simulink model "Code_2DoF_Simulation_myori"  (R2022b)
settings: Solver=ode4  StartTime=0  StopTime=32  FixedStep=0.0025  MaxStep=0.005  MinStep=0.001  RelTol=0.5
settings Model: Creator=hp  LastModifiedBy=33093
settings SolverCC: AlgebraicLoopSolver=TrustRegion
settings DataIOCC: ExternalInput=untitled.getElement(1),[],[],[],[],[],[],[],[],[],[],[],[],[],[],[],[],[],[]  SaveFormat=Array  SignalLoggingSaveFormat=ModelDataLogs  ReturnWorkspaceOutputs=off  SignalLoggingName=sigsOut
settings OptimizationCC: DefaultParameterBehavior=Inlined  UseDivisionForNetSlopeComputation=on  UseFloatMulNetSlope=on  InlineInvariantSignals=on  PassReuseOutputArgsAs=Individual arguments  ExpressionDepthLimit=2147483647  ZeroExternalMemoryAtStartup=off  ZeroInternalMemoryAtStartup=off  NoFixptDivByZeroProtection=on  EfficientFloat2IntCast=on  LifeSpan=1  EfficientTunableParamExpr=on
settings DebuggingCC: SaveWithParameterizedLinksMsg=none  UnderspecifiedInitializationDetection=Classic  MergeDetectMultiDrivingBlocksExec=none  SignalResolutionControl=TryResolveAllWithWarning  MultiTaskDSMMsg=warning  MultiTaskCondExecSysMsg=none  MultiTaskRateTransMsg=warning  ParameterTunabilityLossMsg=error  FcnCallInpInsideContextMsg=warning  UnconnectedInputMsg=warning  UnconnectedOutputMsg=warning  UnconnectedLineMsg=warning  StateNameClashWarn=warning  SFUnexpectedBacktrackingDiag=warning  SFNoUnconditionalDefaultTransitionDiag=warning  SFExecutionAtInitializationDiag=none  SFMachineParentedDataDiag=warning  ArithmeticOperatorsInVariantConditions=warning
settings HardwareCC: TargetBitPerPointer=64  TargetBitPerSizeT=64  TargetBitPerPtrDiffT=64  TargetLongLongMode=on  TargetIntDivRoundTo=Zero  TargetEndianess=LittleEndian  TargetWordSize=64  TargetHWDeviceType=MATLAB Host  ProdEqTarget=off
settings ModelReferenceCC: EnableRefExpFcnMdlSchedulingChecks=on  PropagateSignalLabelsOutOfModel=off
settings SFSimCC: SimUseLocalCustomCode=off  MATLABDynamicMemAlloc=off  CustomCodeUndefinedFunction=UseInterfaceOnly
settings RTWCC: Description=Embedded Coder  SystemTargetFile=ert.tlc  TemplateMakefile=ert_default_tmf  GenerateReport=on  RTWUseLocalCustomCode=off  IncludeHyperlinkInReport=on  LaunchReport=on  GenerateTraceInfo=on  GenerateTraceReport=on  GenerateTraceReportSl=on  GenerateTraceReportSf=on  GenerateTraceReportEml=on  GenerateCodeMetricsReport=on
settings CodeAppCC: ForceParamTrailComments=on  IgnoreCustomStorageClasses=off  MaxIdLength=128  OperatorAnnotations=on  SimulinkDataObjDesc=on  SFDataObjDesc=on  MATLABFcnDesc=on  CustomSymbolStrGlobalVar=rt$N$M  CustomSymbolStrType=$N$M  CustomSymbolStrFcn=$N$M$F  CustomSymbolStrMacro=$N$M  InsertBlockDesc=on  StateflowObjectComments=on  MATLABSourceComments=on
settings ERTTargetCC: MultiwordLength=2048  GenerateSampleERTMain=on  CombineSignalStateStructs=on  SupportComplex=off  SupportNonInlinedSFcns=on  InlinedParameterPlacement=NonHierarchical  ERTCustomFileTemplate=example_file_process.tlc  ERTFilePackagingFormat=CompactWithDataFile
settings ConfigComp: CovMetricSettings=dw  CovSaveCumulativeToWorkspaceVar=on  CovSaveSingleToWorkspaceVar=on  CovExternalEMLEnable=off

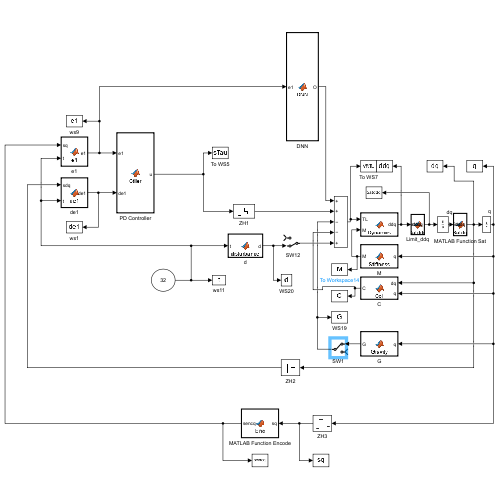
[thumbnail: Simulink's stored preview of the top-level diagram]
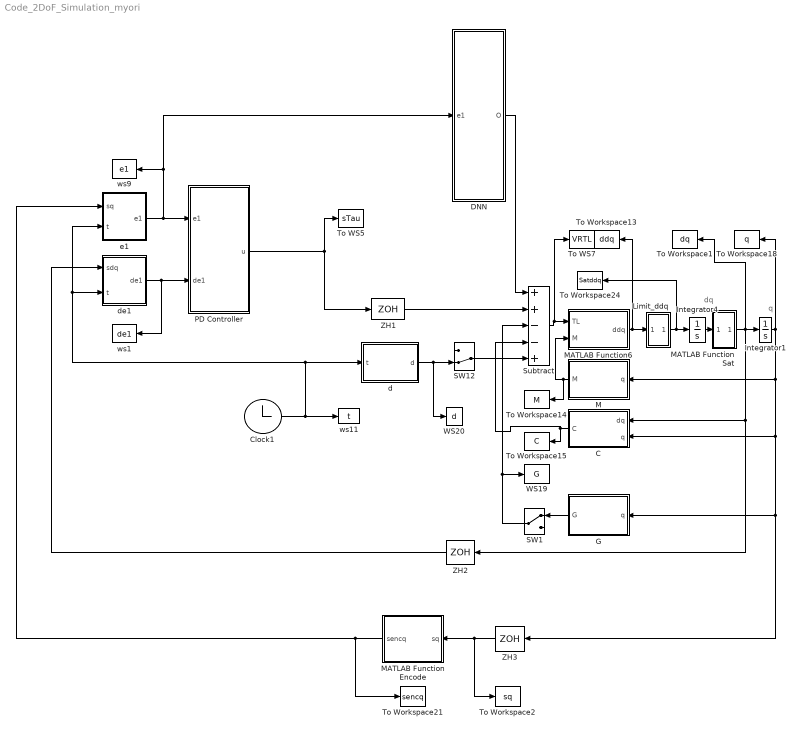
== system Code_2DoF_Simulation_myori ==
  note: q
  note: dq
  C : MATLAB Function  TreatAsAtomicUnit=on
  Clock1 : Clock
  DNN : MATLAB Function  TreatAsAtomicUnit=on
  G : MATLAB Function  TreatAsAtomicUnit=on
  Integrator1 : Integrator  InitialCondition=[-1;0]
  Integrator4 : Integrator  InitialCondition=[0;0]
  Limit_ddq : MATLAB Function  TreatAsAtomicUnit=on
  M : MATLAB Function  TreatAsAtomicUnit=on
  MATLAB Function Encode : MATLAB Function  TreatAsAtomicUnit=on
  MATLAB Function Sat : MATLAB Function  TreatAsAtomicUnit=on
  MATLAB Function6 : MATLAB Function  TreatAsAtomicUnit=on
  PD Controller : MATLAB Function  TreatAsAtomicUnit=on
  SW1 : ManualSwitch
  SW12 : ManualSwitch  CurrentSetting=0
  Subtract : Sum  Inputs=++--+
  To WS5 : ToWorkspace  VariableName=sTau  SampleTime=-1
  To WS7 : ToWorkspace  VariableName=VRTL  SampleTime=-1
  To Workspace1 : ToWorkspace  VariableName=dq  SampleTime=-1
  To Workspace13 : ToWorkspace  VariableName=ddq  SampleTime=-1
  To Workspace14 : ToWorkspace  VariableName=M  SampleTime=-1
  To Workspace15 : ToWorkspace  VariableName=C  SampleTime=-1
  To Workspace18 : ToWorkspace  VariableName=q  SampleTime=-1
  To Workspace2 : ToWorkspace  VariableName=sq  SampleTime=-1
  To Workspace21 : ToWorkspace  VariableName=sencq  SampleTime=-1
  To Workspace24 : ToWorkspace  VariableName=Satddq  SampleTime=-1
  WS19 : ToWorkspace  VariableName=G  SampleTime=-1
  WS20 : ToWorkspace  VariableName=d  SampleTime=-1
  ZH1 : ZeroOrderHold  SampleTime=0.0025
  ZH2 : ZeroOrderHold  SampleTime=0.0025
  ZH3 : ZeroOrderHold  SampleTime=0.0025
  d : MATLAB Function  TreatAsAtomicUnit=on
  de1 : MATLAB Function  TreatAsAtomicUnit=on
  e1 : MATLAB Function  TreatAsAtomicUnit=on
  ws1 : ToWorkspace  VariableName=de1  SampleTime=-1
  ws11 : ToWorkspace  VariableName=t  SampleTime=-1
  ws9 : ToWorkspace  VariableName=e1  SampleTime=-1
  wires:
  MATLAB Function6/1(ddq) -> To Workspace13/1, Limit_ddq/1(ddq)
  SW1/1 -> Subtract/3, WS19/1
  C/1(C) -> Subtract/4, To Workspace15/1
  Subtract/1 -> To WS7/1, MATLAB Function6/1(TL)
  M/1(M) -> MATLAB Function6/2(M), To Workspace14/1
  Integrator1/1 -> ZH3/1, G/1(q), C/2(q), M/1(q), To Workspace18/1
  ZH1/1 -> Subtract/2
  Clock1/1 -> ws11/1, e1/2(t), de1/2(t), d/1(t)
  ZH3/1 -> MATLAB Function Encode/1(sq), To Workspace2/1
  Integrator4/1 -> MATLAB Function Sat/1(dq)
  MATLAB Function Sat/1(Satdq) -> To Workspace1/1, ZH2/1, C/1(dq), Integrator1/1
  Limit_ddq/1(Satddq) -> To Workspace24/1, Integrator4/1
  de1/1(de1) -> ws1/1, PD Controller/2(de1)
  ZH2/1 -> de1/1(sdq)
  MATLAB Function Encode/1(sencq) -> To Workspace21/1, e1/1(sq)
  d/1(d) -> WS20/1, SW12/2
  SW12/1 -> Subtract/5
  PD Controller/1(u) -> ZH1/1, To WS5/1
  G/1(G) -> SW1/1
  DNN/1(O) -> Subtract/1
  e1/1(e1) -> PD Controller/1(e1), DNN/1(e1), ws9/1

== matlab function Code_2DoF_Simulation_myori/MATLAB Function Encode ==
  settings: updateMethod=DISCRETE  sampleTime=0.0025
  data: sq input; sencq output
function sencq = Enc(sq)
Delta=2*pi/2^19;
sencq=[0;0];
for i=1:1:2
    Number=floor(sq(i)/Delta)+1;
    sencq(i)=Number*Delta;
end
sencq=[sencq(1);sencq(2)];
% sencq=[sq(1);sq(2)];
end

== matlab function Code_2DoF_Simulation_myori/PD Controller ==
  settings: updateMethod=DISCRETE  sampleTime=0.0025
  data: e1 input; de1 input; u output
function u = Ctller(e1,de1)
% kp1=5000; kp2=1000; kd1=1000; kd2=80;
kp1=1000; kp2=800; kd1=500; kd2=80;
Kp=diag([kp1;kp2]);Kd=diag([kd1;kd2]);
u=-Kp*e1-Kd*de1;
end

== matlab function Code_2DoF_Simulation_myori/de1 ==
  settings: updateMethod=DISCRETE  sampleTime=0.0025
  data: sdq input; t input; de1 output
function de1 = de1(sdq,t)
dqd1=pi/4*cos(pi/4*t);
dqd2=pi/2*sin(pi/4*(t+pi/2))*-pi/8*sin(pi/8*(t+pi/2))+pi/2*cos(pi/8*(t+pi/2))*pi/4*cos(pi/4*(t+pi/2));
% dqd1=0;
% dqd2=0;
dqd=[dqd1;dqd2];
de1=sdq-dqd;
end

== matlab function Code_2DoF_Simulation_myori/Limit_ddq ==
  settings: updateMethod=CONTINUOUS
  data: ddq input; Satddq output
function Satddq = Satddq(ddq)
Amax=10000*pi/2;   % 10000
for i=1:1:2
    if ddq(i)>Amax
        ddq(i)=Amax;
    elseif ddq(i)<-Amax
        ddq(i)=-Amax;
    end
end
Satddq=[ddq(1);ddq(2)];
end

== matlab function Code_2DoF_Simulation_myori/DNN ==
  settings: updateMethod=DISCRETE  sampleTime=0.0025
  data: e1 input; O output; o_py parameter double
function O = DNN(e1,o_py)
O=o_py;
end

== matlab function Code_2DoF_Simulation_myori/G ==
  settings: updateMethod=CONTINUOUS  sampleTime=0.0005
  data: q input; G output
function G = Gravity(q)
q1=q(1);q2=q(2);
s1=sin(q1);s2=sin(q2);
c1=cos(q1);c2=cos(q2);
c12=cos(q1+q2);
m1=5;m2=5;
l1=1;l2=1;
g=9.81;
G1 = m1*g*l1*c1/2+m2*g*l1*c1+m2*g*l2*c12/2; 
G2 = m2*g*l2*c12/2;
G=[G1;
   G2]; 
end

== matlab function Code_2DoF_Simulation_myori/C ==
  settings: updateMethod=CONTINUOUS  sampleTime=0.0005
  data: dq input; C output; q input
function C = Col(dq,q)
q1=q(1);q2=q(2);
dq1=dq(1);dq2=dq(2);
s1=sin(q1);s2=sin(q2);
c1=cos(q1);c2=cos(q2);
m1=5;m2=5;
l1=1;l2=1;
g=9.81;
C11=-m2*l1*l2*s2*dq2;
C12=-m2*l1*l2*s2*dq2/2;
C21=m2*l1*l2*s2*dq1/2;
C22=0;
CM=[C11 C12
    C21 C22];
C=CM*dq;
end

== matlab function Code_2DoF_Simulation_myori/e1 ==
  settings: updateMethod=DISCRETE  sampleTime=0.0025
  data: sq input; e1 output; t input
function e1 = e1(sq,t)
q=[sq(1);sq(2)];
qd1=sin(pi/4*t)-pi/2;
qd2=pi/2*cos(pi/8*(t+pi/2))*sin(pi/4*(t+pi/2));
% qd1=1;
% qd2=1;
qd=[qd1;qd2]; 
e1=q-qd;
end

== matlab function Code_2DoF_Simulation_myori/MATLAB Function6 ==
  settings: updateMethod=CONTINUOUS  sampleTime=0.0005
  data: TL input; M input; ddq output
function ddq = Dynamics(TL,M)

M22 = [M(1) M(2)
       M(3) M(4)];
ddq=M22 \ TL;
end

== matlab function Code_2DoF_Simulation_myori/M ==
  settings: updateMethod=CONTINUOUS  sampleTime=0.0005
  data: q input; M output
function M = Stiffness(q)
q1=q(1);q2=q(2);
s1=sin(q1);s2=sin(q2);
c1=cos(q1);c2=cos(q2);
m1=5;m2=5;
l1=1;l2=1;
g=9.81;
M11=m1*l1^2/3+m2*l1^2+m2*l2^2/4+m2*l1*l2*c2;
M12=m2*l2^2/4+m2*l1*l2*c2/2;
M22=m2*l2^2/3;
M = [M11; M12; 
     M12; M22];
end

== matlab function Code_2DoF_Simulation_myori/MATLAB Function Sat ==
  settings: updateMethod=CONTINUOUS
  data: dq input; Satdq output
function Satdq = Satdq(dq)
Vmax=2000;
for i=1:1:2
    if dq(i)>Vmax
        dq(i)=Vmax;
    elseif dq(i)<-Vmax
        dq(i)=-Vmax;
    end
end
Satdq=[dq(1);dq(2)];
end

== matlab function Code_2DoF_Simulation_myori/d ==
  settings: updateMethod=CONTINUOUS  sampleTime=0.0005
  data: t input; d output
function d = disturbance(t)
if t>10
% d=0.1*rand(6,1);
d=50.0*[sin(0.6*(t-10));sin(0.6*(t-10))];
else
    d=zeros(2,1);
% d=0.1*rand(6,1)*3*sin(0.5*t);
% d=0.3*sin(0.5*t)*ones(6,1);
end
end
